simulink model "Systems"  (R2022b)
settings: Solver=VariableStepAuto  StartTime=0.0  StopTime=10.0  RelTol=1e-3
settings Model: Creator=brbar  LastModifiedBy=brbar

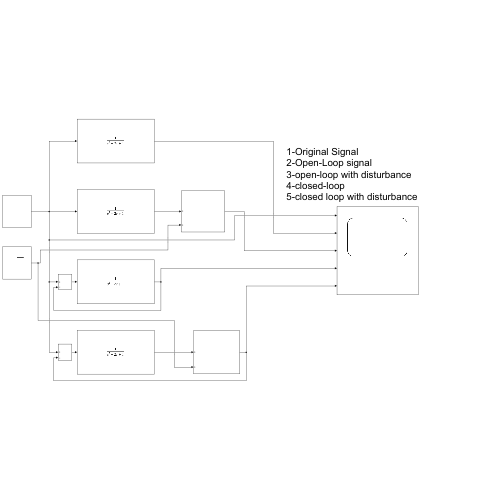
[thumbnail: Simulink's stored preview of the top-level diagram]
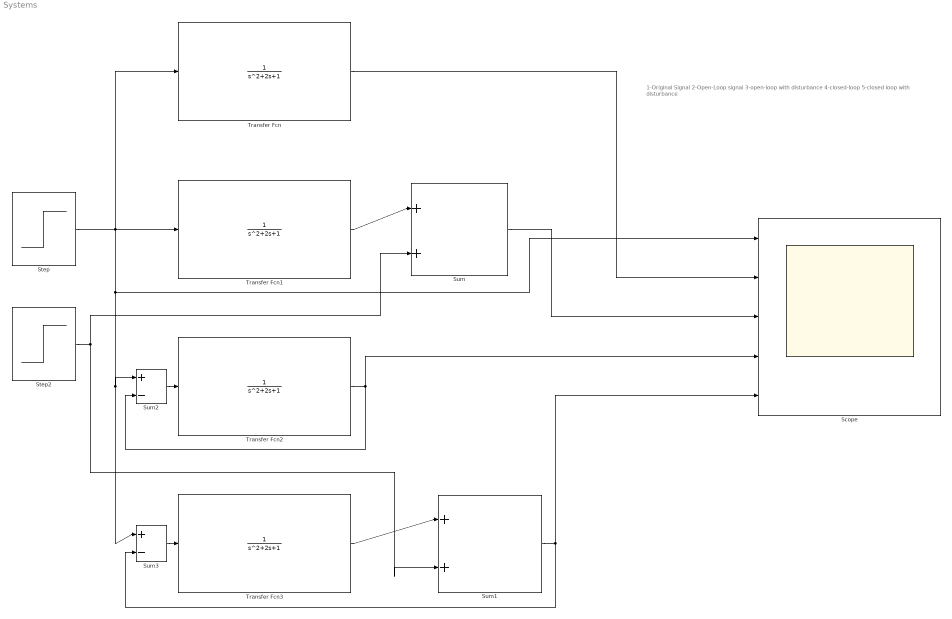
== system Systems ==
  note: 1-Original Signal
      | 2-Open-Loop signal
      | 3-open-loop with disturbance
      | 4-closed-loop
      | 5-closed loop with disturbance
  Scope : Scope  NumInputPorts=5
  Step : Step  SampleTime=0
  Step2 : Step  Time=2  After=0.3  SampleTime=0
  Sum : Sum  Inputs=|++
  Sum1 : Sum  Inputs=|++
  Sum2 : Sum  Inputs=|+-
  Sum3 : Sum  Inputs=|+-
  Transfer Fcn{,1..3} (4 alike) : TransferFcn
  wires:
  Step/1 -> Transfer Fcn1/1, Transfer Fcn/1, Scope/1, Sum3/1, Sum2/1
  Sum2/1 -> Transfer Fcn2/1
  Sum3/1 -> Transfer Fcn3/1
  Transfer Fcn2/1 -> Scope/4, Sum2/2
  Transfer Fcn3/1 -> Sum1/1
  Sum1/1 -> Scope/5, Sum3/2
  Transfer Fcn1/1 -> Sum/1
  Step2/1 -> Sum1/2, Sum/2
  Sum/1 -> Scope/3
  Transfer Fcn/1 -> Scope/2
